simulink model "Multiple_MPC_Controller"  (R2024b)
settings: configuration reference "controller_config" (kept outside this file)
libraries: mpclib x1
settings Model: DataDictionary=sim_data_vehicle.sldd  Creator=tshintai  LastModifiedBy=tshintai
settings ConfigSetRef: SourceName=controller_config

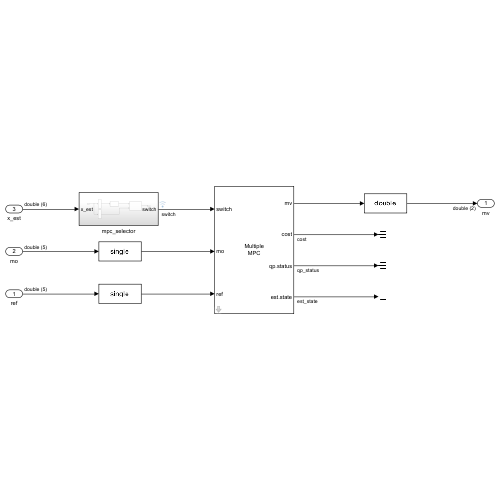
[thumbnail: Simulink's stored preview of the top-level diagram]
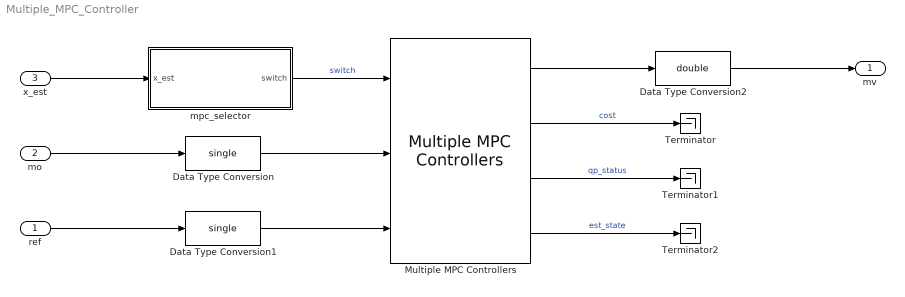
== system Multiple_MPC_Controller ==
  ref : Inport  OutDataTypeStr=double  PortDimensions=5
  mo : Inport  Port=2  OutDataTypeStr=double  PortDimensions=5
  x_est : Inport  Port=3  OutDataTypeStr=double  PortDimensions=6
  Data Type Conversion : DataTypeConversion  OutDataTypeStr=single  SaturateOnIntegerOverflow=off  RndMeth=Floor
  Data Type Conversion1 : DataTypeConversion  OutDataTypeStr=single  SaturateOnIntegerOverflow=off  RndMeth=Floor
  Data Type Conversion2 : DataTypeConversion  OutDataTypeStr=double  SaturateOnIntegerOverflow=off  RndMeth=Floor
  Multiple MPC Controllers : mpclib/Multiple MPC Controllers  mpcobjs=mpcObj_multi  x0s=x0_multi  Nmpc=1  theMPC=1  nmv=1  nmo=1  nmd=1  nts=1  md_inport_multiple=off  mv_inport_multiple=off  uref_inport_multiple=off  return_cost_multiple=on  return_mvseq_multiple=off  return_qpstatus_multiple=on  return_xseq_multiple=off  return_state_multiple=on  return_ovseq_multiple=off  state_inport_multiple=off  umin_inport_multiple=off  umax_inport_multiple=off  ymin_inport_multiple=off  ymax_inport_multiple=off  ywt_inport_multiple=off  uwt_inport_multiple=off  duwt_inport_multiple=off  rhoeps_inport_multiple=off  BlockDataType_multiple=single  SampleTimeInherited_multiple=off
  Terminator : Terminator
  Terminator1 : Terminator
  Terminator2 : Terminator
  mpc_selector : Subsystem
  mv : Outport  OutDataTypeStr=double  PortDimensions=2
  wires:
  Multiple MPC Controllers/3 -> Terminator1/1  "qp_status"
  Multiple MPC Controllers/4 -> Terminator2/1  "est_state"
  Multiple MPC Controllers/1 -> Data Type Conversion2/1
  mpc_selector/1(switch) -> Multiple MPC Controllers/1  "switch"
  Data Type Conversion2/1 -> mv/1
  Data Type Conversion1/1 -> Multiple MPC Controllers/3
  ref/1 -> Data Type Conversion1/1
  Data Type Conversion/1 -> Multiple MPC Controllers/2
  x_est/1 -> mpc_selector/1(x_est)
  Multiple MPC Controllers/2 -> Terminator/1  "cost"
  mo/1 -> Data Type Conversion/1

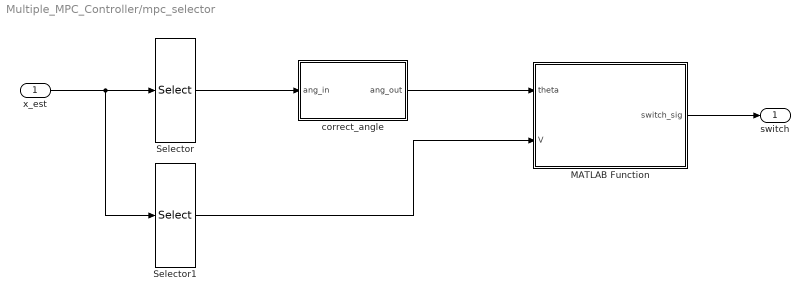
== system Multiple_MPC_Controller/mpc_selector ==
  x_est : Inport
  MATLAB Function : MATLAB Function  TreatAsAtomicUnit=on
  Selector : Selector  InputPortWidth=6  IndexOptions=Index vector (dialog)  Indices=[3]  OutputSizes=1
  Selector1 : Selector  InputPortWidth=6  IndexOptions=Index vector (dialog)  Indices=[6]  OutputSizes=1
  correct_angle : Subsystem
  switch : Outport
  wires:
  MATLAB Function/1(switch_sig) -> switch/1
  Selector/1 -> correct_angle/1(ang_in)
  x_est/1 -> Selector1/1, Selector/1
  Selector1/1 -> MATLAB Function/2(V)
  correct_angle/1(ang_out) -> MATLAB Function/1(theta)

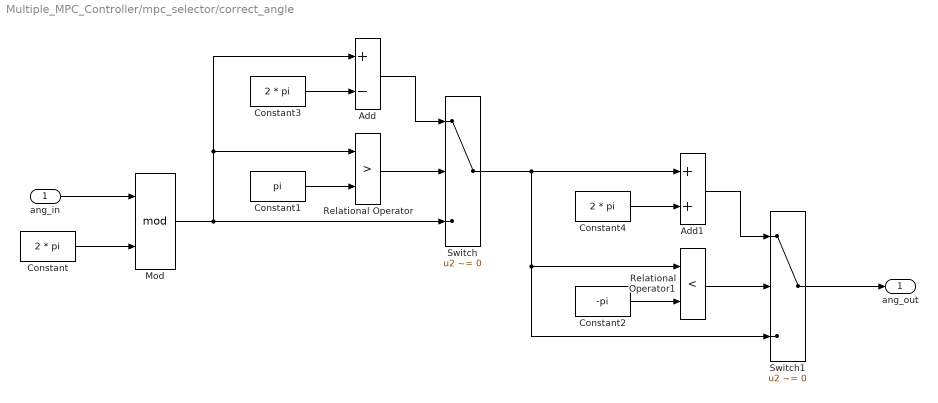
== system Multiple_MPC_Controller/mpc_selector/correct_angle ==
  ang_in : Inport
  Add : Sum  Inputs=+-
  Add1 : Sum
  Constant : Constant  Value=2 * pi
  Constant1 : Constant  Value=pi
  Constant2 : Constant  Value=-pi
  Constant3 : Constant  Value=2 * pi
  Constant4 : Constant  Value=2 * pi
  Mod : Math  Operator=mod
  Relational Operator : RelationalOperator  Operator=>  OutDataTypeStr=boolean  RndMeth=Simplest  InputSameDT=off
  Relational Operator1 : RelationalOperator  Operator=<  OutDataTypeStr=boolean  RndMeth=Simplest  InputSameDT=off
  Switch : Switch  Criteria=u2 ~= 0  SaturateOnIntegerOverflow=off  InputSameDT=off
  Switch1 : Switch  Criteria=u2 ~= 0  SaturateOnIntegerOverflow=off  InputSameDT=off
  ang_out : Outport
  wires:
  Relational Operator/1 -> Switch/2
  Switch/1 -> Switch1/3, Relational Operator1/1, Add1/1
  Mod/1 -> Switch/3, Add/1, Relational Operator/1
  Switch1/1 -> ang_out/1
  Constant/1 -> Mod/2
  Constant1/1 -> Relational Operator/2
  Add/1 -> Switch/1
  ang_in/1 -> Mod/1
  Constant3/1 -> Add/2
  Constant4/1 -> Add1/2
  Add1/1 -> Switch1/1
  Constant2/1 -> Relational Operator1/2
  Relational Operator1/1 -> Switch1/2

== matlab function Multiple_MPC_Controller/mpc_selector/MATLAB Function ==
  data: theta input; switch_sig output; V input; op_pattern_mat parameter
function switch_sig = select_MPC(theta, V, op_pattern_mat)

dist_vec = zeros(size(op_pattern_mat, 2), 1);

for i = 1:size(dist_vec, 1)
    
    theta_comp = theta - op_pattern_mat(1, i);
    if (theta_comp > pi)
        theta_comp = theta_comp - 2 * pi;
    elseif (theta_comp < -pi)
        theta_comp = theta_comp + 2 * pi;
    end
    
    dist_vec(i) = theta_comp ^ 2 + (V - op_pattern_mat(2, i)) ^ 2;
end

[~, idx] = min(dist_vec);

switch_sig = int32(idx);

end
